simulink model "forcesandtorques_model"  (Simulink 7.7)
settings: Solver=ode45  StartTime=0.0  StopTime=10.0  RelTol=1e-3
settings Model: Creator=Administrator  LastModifiedBy=Administrator

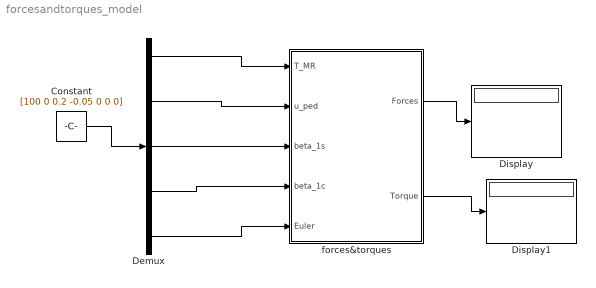
== system forcesandtorques_model ==
  Constant : Constant  Value=[100 0 0.2 -0.05 0 0 0]
  Demux : Demux  Outputs=[1 1 1 1 3]
  Display : Display
  Display1 : Display
  forces&torques : Subsystem  mask{mass0=44.384, AQ=0.00036, BQ=0.01, lm=0, ym=0, hm=0, Lt=1.2, Ht=0.2}
  wires:
  forces&torques/1(Forces) -> Display/1
  forces&torques/2(Torque) -> Display1/1
  Demux/1 -> forces&torques/1(T_MR)
  Demux/2 -> forces&torques/2(u_ped)
  Demux/3 -> forces&torques/3(beta_1s)
  Demux/4 -> forces&torques/4(beta_1c)
  Demux/5 -> forces&torques/5(Euler)
  Constant/1 -> Demux/1

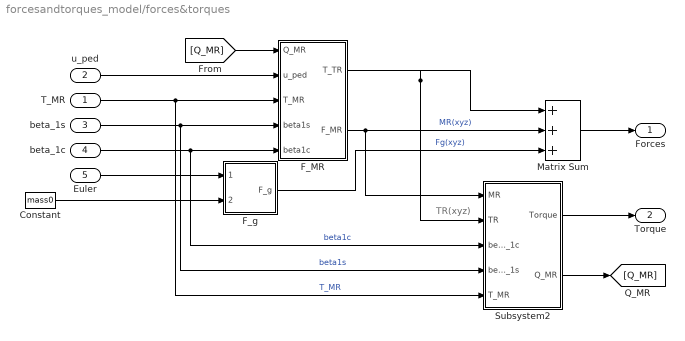
== system forcesandtorques_model/forces&torques ==
  note: TR(xyz)
  T_MR : Inport
  u_ped : Inport  Port=2
  beta_1s : Inport  Port=3
  beta_1c : Inport  Port=4
  Euler : Inport  Port=5
  Constant : Constant  Value=mass0
  F_MR : Subsystem
  F_g : Subsystem
  Matrix Sum : Sum  Inputs=+++  CollapseMode=Specified dimension  CollapseDim=3
  Subsystem2 : Subsystem
  Forces : Outport
  Torque : Outport  Port=2
  wires:
  F_MR/1(T_TR) -> Subsystem2/2(TR), Matrix Sum/1
  u_ped/1 -> F_MR/2(u_ped)
  Matrix Sum/1 -> Forces/1
  Subsystem2/1(Torque) -> Torque/1
  Constant/1 -> F_g/2(mass)
  F_g/1(F_g) -> Matrix Sum/3  "Fg(xyz)"
  F_MR/2(F_MR) -> Subsystem2/1(MR), Matrix Sum/2  "MR(xyz)"
  Euler/1 -> F_g/1(Euler)
  T_MR/1 -> Subsystem2/5(T_MR), F_MR/3(T_MR)  "T_MR"
  beta_1c/1 -> Subsystem2/3(beta_1c), F_MR/5(beta1c)  "beta1c"
  beta_1s/1 -> Subsystem2/4(beta_1s), F_MR/4(beta1s)  "beta1s"
  Subsystem2/2(Q_MR) -> [Q_MR]
  [Q_MR] -> F_MR/1(Q_MR)

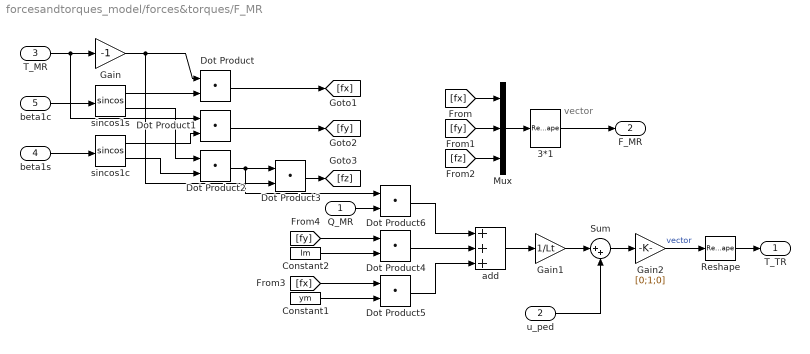
== system forcesandtorques_model/forces&torques/F_MR ==
  note: vector
  Q_MR : Inport
  u_ped : Inport  Port=2
  T_MR : Inport  Port=3
  beta1s : Inport  Port=4
  beta1c : Inport  Port=5
  3*1 : Reshape  OutputDimensionality=Column vector (2-D)
  Constant1 : Constant  Value=ym
  Constant2 : Constant  Value=lm
  Dot Product{,1..6} (7 alike) : DotProduct  InputSameDT=on  OutDataTypeStr=Inherit: Inherit via internal rule
  Gain : Gain  Gain=-1
  Gain1 : Gain  Gain=1/Lt
  Gain2 : Gain  Gain=[0;1;0]
  Mux : Mux  Inputs=3
  Reshape : Reshape  OutputDimensionality=Column vector (2-D)
  Sum : Sum  Inputs=|++
  add : Sum  Inputs=+++
  sincos1c : Trigonometry  Operator=sincos
  sincos1s : Trigonometry  Operator=sincos
  T_TR : Outport
  F_MR : Outport  Port=2
  wires:
  u_ped/1 -> Sum/2
  Gain1/1 -> Sum/1
  add/1 -> Gain1/1
  Q_MR/1 -> Dot Product6/2
  Constant1/1 -> Dot Product5/2
  Constant2/1 -> Dot Product4/2
  3*1/1 -> F_MR/1
  Mux/1 -> 3*1/1
  beta1s/1 -> sincos1c/1
  beta1c/1 -> sincos1s/1
  Dot Product2/1 -> Dot Product6/1, Dot Product3/1
  sincos1c/2 -> Dot Product2/2
  sincos1s/2 -> Dot Product2/1
  sincos1c/1 -> Dot Product1/2
  sincos1s/1 -> Dot Product/2
  Gain/1 -> Dot Product3/2, Dot Product/1
  T_MR/1 -> Gain/1, Dot Product1/1
  Dot Product/1 -> [fx]
  Dot Product1/1 -> [fy]
  Dot Product3/1 -> [fz]
  [fx] -> Mux/1
  [fy] -> Mux/2
  [fz] -> Mux/3
  [fy] -> Dot Product4/1
  [fx] -> Dot Product5/1
  Dot Product6/1 -> add/1
  Dot Product4/1 -> add/2
  Dot Product5/1 -> add/3
  Sum/1 -> Gain2/1
  Gain2/1 -> Reshape/1  "vector"
  Reshape/1 -> T_TR/1

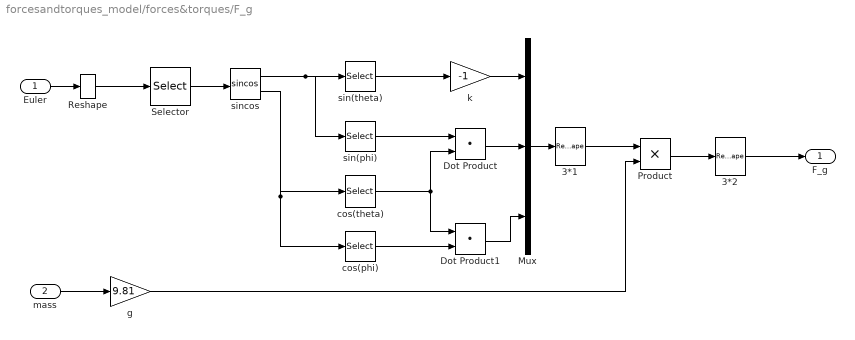
== system forcesandtorques_model/forces&torques/F_g ==
  Euler : Inport
  mass : Inport  Port=2  PortDimensions=1
  3*1 : Reshape  OutputDimensionality=Column vector (2-D)
  3*2 : Reshape  OutputDimensionality=Column vector (2-D)
  Dot Product : DotProduct  InputSameDT=on  OutDataTypeStr=Inherit: Inherit via internal rule
  Dot Product1 : DotProduct  InputSameDT=on  OutDataTypeStr=Inherit: Inherit via internal rule
  Mux : Mux  Inputs=3
  Product : Product  RndMeth=Zero
  Reshape : Reshape  OutputDimensionality=Column vector (2-D)
  Selector : Selector  InputPortWidth=3  IndexOptions=Index vector (dialog)  Indices=[1 2]  OutputSizes=1
  cos(phi) : Selector  InputPortWidth=2  IndexOptions=Index vector (dialog)  Indices=[1]  OutputSizes=1
  cos(theta) : Selector  InputPortWidth=2  IndexOptions=Index vector (dialog)  Indices=[2]  OutputSizes=1
  g : Gain  Gain=9.81
  k : Gain  Gain=-1
  sin(phi) : Selector  InputPortWidth=2  IndexOptions=Index vector (dialog)  Indices=[1]  OutputSizes=1
  sin(theta) : Selector  InputPortWidth=2  IndexOptions=Index vector (dialog)  Indices=[2]  OutputSizes=1
  sincos : Trigonometry  Operator=sincos
  F_g : Outport
  wires:
  cos(phi)/1 -> Dot Product1/2
  Reshape/1 -> Selector/1
  Euler/1 -> Reshape/1
  mass/1 -> g/1
  Dot Product1/1 -> Mux/3
  Dot Product/1 -> Mux/2
  cos(theta)/1 -> Dot Product1/1, Dot Product/2
  sin(phi)/1 -> Dot Product/1
  k/1 -> Mux/1
  sin(theta)/1 -> k/1
  sincos/2 -> cos(theta)/1, cos(phi)/1
  sincos/1 -> sin(theta)/1, sin(phi)/1
  Selector/1 -> sincos/1
  Mux/1 -> 3*1/1
  3*1/1 -> Product/1
  g/1 -> Product/2
  Product/1 -> 3*2/1
  3*2/1 -> F_g/1

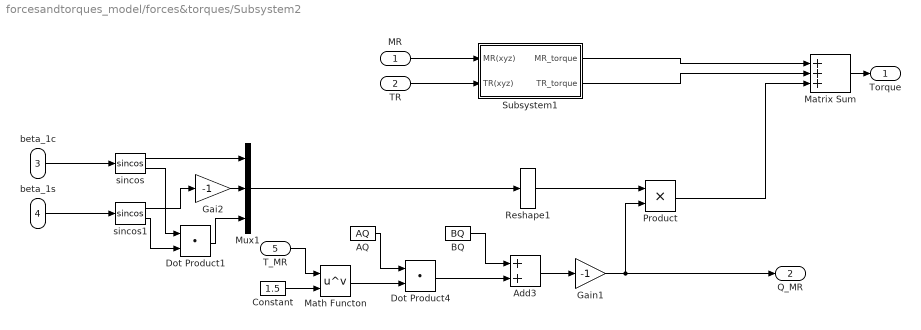
== system forcesandtorques_model/forces&torques/Subsystem2 ==
  MR : Inport  PortDimensions=3
  TR : Inport  Port=2  PortDimensions=3
  beta_1c : Inport  Port=3  PortDimensions=1
  beta_1s : Inport  Port=4  PortDimensions=1
  T_MR : Inport  Port=5
  AQ : Constant  Value=AQ
  Add3 : Sum
  BQ : Constant  Value=BQ  VectorParams1D=off
  Constant : Constant  Value=1.5
  Dot Product1 : DotProduct  InputSameDT=on  OutDataTypeStr=Inherit: Inherit via internal rule
  Dot Product4 : DotProduct  InputSameDT=on  OutDataTypeStr=Inherit: Inherit via internal rule
  Gai2 : Gain  Gain=-1
  Gain1 : Gain  Gain=-1
  Math Functon : Math  Operator=pow  SaturateOnIntegerOverflow=on
  Matrix Sum : Sum  Inputs=+++  CollapseMode=Specified dimension  CollapseDim=3
  Mux1 : Mux  Inputs=3
  Product : Product  RndMeth=Zero
  Reshape1 : Reshape  OutputDimensionality=Column vector (2-D)
  Subsystem1 : Subsystem
  sincos : Trigonometry  Operator=sincos
  sincos1 : Trigonometry  Operator=sincos
  Torque : Outport
  Q_MR : Outport  Port=2
  wires:
  T_MR/1 -> Math Functon/1
  Matrix Sum/1 -> Torque/1
  beta_1s/1 -> sincos1/1
  beta_1c/1 -> sincos/1
  TR/1 -> Subsystem1/2(TR(xyz))
  MR/1 -> Subsystem1/1(MR(xyz))
  Subsystem1/2(TR_torque) -> Matrix Sum/2
  Subsystem1/1(MR_torque) -> Matrix Sum/1
  Gain1/1 -> Q_MR/1, Product/2
  Dot Product1/1 -> Mux1/3
  sincos/2 -> Dot Product1/1
  sincos1/2 -> Dot Product1/2
  Gai2/1 -> Mux1/2
  sincos1/1 -> Gai2/1
  sincos/1 -> Mux1/1
  Add3/1 -> Gain1/1
  Dot Product4/1 -> Add3/2
  BQ/1 -> Add3/1
  AQ/1 -> Dot Product4/1
  Math Functon/1 -> Dot Product4/2
  Constant/1 -> Math Functon/2
  Product/1 -> Matrix Sum/3
  Mux1/1 -> Reshape1/1
  Reshape1/1 -> Product/1

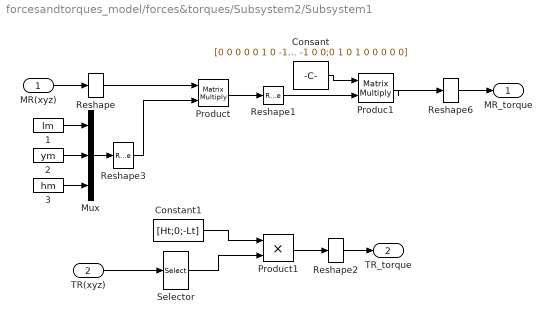
== system forcesandtorques_model/forces&torques/Subsystem2/Subsystem1 ==
  MR(xyz) : Inport
  TR(xyz) : Inport  Port=2
  1 : Constant  Value=lm
  2 : Constant  Value=ym
  3 : Constant  Value=hm
  Consant : Constant  Value=[0 0 0 0 0 1 0 -1 0;0 0 -1 0 0 0 -1 0 0;0 1 0 1 0 0 0 0 0]
  Constant1 : Constant  Value=[Ht;0;-Lt]
  Mux : Mux  Inputs=3
  Produc1 : Product  Multiplication=Matrix(*)  RndMeth=Zero
  Product : Product  Multiplication=Matrix(*)  RndMeth=Zero
  Product1 : Product  RndMeth=Zero
  Reshape{,1..2,6} (4 alike) : Reshape  OutputDimensionality=Column vector (2-D)
  Reshape3 : Reshape  OutputDimensionality=Row vector (2-D)
  Selector : Selector  InputPortWidth=3  IndexOptions=Index vector (dialog)  Indices=[2]  OutputSizes=1
  MR_torque : Outport
  TR_torque : Outport  Port=2
  wires:
  Reshape6/1 -> MR_torque/1
  Produc1/1 -> Reshape6/1
  Consant/1 -> Produc1/1
  Reshape1/1 -> Produc1/2
  TR(xyz)/1 -> Selector/1
  Product/1 -> Reshape1/1
  Reshape3/1 -> Product/2
  Reshape/1 -> Product/1
  Mux/1 -> Reshape3/1
  MR(xyz)/1 -> Reshape/1
  3/1 -> Mux/3
  2/1 -> Mux/2
  1/1 -> Mux/1
  Product1/1 -> Reshape2/1
  Reshape2/1 -> TR_torque/1
  Constant1/1 -> Product1/1
  Selector/1 -> Product1/2
